simulink library "ACCUMULATORS"  (R2019a)
settings: Solver=VariableStepAuto  StartTime=0.0  StopTime=10.0  RelTol=1e-3
libraries: xbsIndex_r4 x1
settings Model: Creator=mybur  LastModifiedBy=mybur

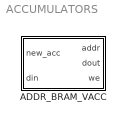
== system ACCUMULATORS ==
  ADDR_BRAM_VACC : Subsystem  mask{vector_length=16, output_sign="SIGNED", output_bit_w=32, output_bin_pt=0}
      mask prompts: vector_length "Vector length"; output_sign "Signed (output)"; output_bit_w "Bitwidth (output)"; output_bin_pt "Binarary point (output)"
      mask init:
      | Simulink.Block.eval([gcb, '/addr_bram_vacc']);
      mask TypeOptions output_sign: "SIGNED" | "UNSIGNED"
      mask DialogControl DescTextVar Prompt: This simple vector accumulator is based on a shift register. It outputs its previous accumulated vector after a new_acc pulse is received.

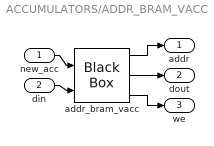
== system ACCUMULATORS/ADDR_BRAM_VACC ==
  new_acc : Inport
  din : Inport  Port=2
  addr_bram_vacc : xbsIndex_r4/Black Box  init_code=addr_bram_vacc_config  sim_method=ISE Simulator  verbose=off  block_type=blackbox2
  addr : Outport
  dout : Outport  Port=2
  we : Outport  Port=3
  wires:
  din/1 -> addr_bram_vacc/2
  new_acc/1 -> addr_bram_vacc/1
  addr_bram_vacc/3 -> we/1
  addr_bram_vacc/1 -> addr/1
  addr_bram_vacc/2 -> dout/1
